simulink library "casper_library"  (Simulink 6.2)
PostLoadFcn:
  | % Stub definitions for mask variables
  | delay_depth=16;
  | n_bits=8;
  | bin_pt=7;
values from neighbouring files (symbols this model uses):
  add_latency = get_var('add_latency', 'defaults', defaults, varargin{:})    [biplex_core_init.m]    (also in butterfly_direct_init.m; dec_fir_init.m = get_var('add_latency','defaults', defaults, varargin{:}); fft_biplex_real_4x_init.m; fft_direct_init.m)
  BitWidth = get_var('BitWidth', 'defaults', defaults, varargin{:})    [biplex_core_init.m]    (also in butterfly_direct_init.m; fft_biplex_init.m; fft_biplex_real_2x_init.m; fft_biplex_real_4x_init.m)
  blockCountBits = ceil(log2(numBlocks))    [address_gen_vacc_v2_mask.m]
  blockRowBits = 0    [address_gen_vacc_v2_mask.m]
  mult_latency = get_var('mult_latency', 'defaults', defaults, varargin{:})    [biplex_core_init.m]    (also in butterfly_direct_init.m; dec_fir_init.m = get_var('mult_latency','defaults', defaults, varargin{:}); fft_biplex_real_4x_init.m; fft_direct_init.m)
  n_inputs = get_var('n_inputs', 'defaults', defaults, varargin{:})    [adder_tree_init.m]    (also in barrel_switcher_init.m; dec_fir_init.m = get_var('n_inputs','defaults', defaults, varargin{:}); fft_init.m; fft_unscrambler_init.m)
undefined symbols (not defined in the file or in its folder): acc_len, ant_bits, bit_growth, bit_rev, BitWidthIn, cmult_4bit_br, cmult_4bit_em, cmult_4bit_sl, CoeffBitWidth, DelayLen, n_ants, n_bits_out, pfb_coeff_gen_calc, PFBSize
libraries: xbsIndex_r3 x2630, casper_library x215, xps_library x24, fft_library x4
(part 3 of 21)

== system casper_library/Delays/delay_bram_prog_dp ==
  din : Inport  Port=1  LatchInput=off
  delay : Inport  Port=2  LatchInput=off
  AddSub : xbsIndex_r3/AddSub  mode=Subtraction  precision=User Defined  arith_type=Unsigned  n_bits=ram_bits  bin_pt=0  quantization=Truncate  overflow=Wrap  latency=1  explicit_period=off  period=1  use_carryin=off  use_carryout=off  en=off  dbl_ovrd=off  show_param=off  use_core=on  pipeline=off  use_rpm=on  gen_core=off
      settings: xl_area=[0, 0, 0, 0, 0, 0, 0]
  Constant2 : xbsIndex_r3/Constant  const=1  equ=P=C  arith_type=Boolean  n_bits=1  bin_pt=0  opselect=C  inp2=PCIN>>17  opr=+  inp1=P  carry=CIN  iostate=0  explicit_period=on  period=1  dbl_ovrd=off
  Constant4 : xbsIndex_r3/Constant  const=0  equ=P=C  arith_type=Boolean  n_bits=1  bin_pt=0  opselect=C  inp2=PCIN>>17  opr=+  inp1=P  carry=CIN  iostate=0  explicit_period=on  period=1  dbl_ovrd=off
  Dual Port RAM : S-Function  AncestorBlock=xbsIndex_r3/Dual Port RAM  FunctionName=xldpram  Parameters=sfcn_mwsv__  mask(Xilinx Dual Port Random Access Memory){depth=2^ram_bits, initVector=0, write_mode_A=Read After Write, write_mode_B=Read After Write, latency=bram_latency, mem_collision=off, init_zero=on, explicit_period=off, period=1, dbl_ovrd=off, rst_a=off, init_a=0, rst_b=off, init_b=0, show_param=off, distributed_mem=off, use_rpm=off, gen_core=off, xl_area=[0, 0, 0, 0, 0, 0, 0], xl_use_area=off}
      mask prompts: initVector "Initial Value Vector"; write_mode_A "Write Mode:  Port A"; write_mode_B "Write Mode:  Port B"; mem_collision "Provide Output Valid Port"; init_zero "Zero Initial Output  (otherwise NaN)"; explicit_period "Use Explicit Sample Period"; period "Sample Period  (use -1 to inherit first known input period)"; dbl_ovrd "Override with Doubles"; rst_a "Provide Reset Port for Port A Output Register"; init_a "Initial Value for Port A Output Register"; rst_b "Provide Reset Port for Port B Output Register"; init_b "Initial Value for Port B Output Register"; show_param "---------------------- Show Implementation Parameters -----------------------------------------------------------------------------------"; distributed_mem "Use Distributed Memory (instead of block RAM)"; use_rpm "Use Placement Information for Core"; gen_core "Generate Core"; xl_area "FPGA Area [Slices, FFs, BRAMs, LUTs, IOBs, Emb. Mults, TBUFs]"; xl_use_area "Use Area Above For Estimation"
      mask help: Dual port random access memory (RAM). Independent address, data and write enable ports allow shared access to a single memory space. Dual ports enable simultaneous access to the memory space at different sample rates using multiple data widths.
      mask init:
      | [designRoot, family, part, speed, package, simulinkPeriod, sysclkPeriod, dbl_ovrd, trimVbit] = xlSysgenSettings(gcb,1,1);
      | if isempty(family)
      | 	family = 'Virtex2';
      | end;
      | dbl_ovrdStr = '';
      | [bg,fg] = xlcmap('XBlock',dbl_ovrd);
      | iPos = get_param(gcb,'Position');
      | iWidth=iPos(3)-iPos(1); iHeight=iPos(4)-iPos(2);
      | iCx=iWidth/2;
      | iCy=iHeight/2;
      | [logoX, logoY] = xlogo(iPos);
      | [memX,memY] = memplot(iPos,min(depth,floor(iWidth/4)));
      | 
      | dataBPNum = 1;
      | dataBStr = '';
      | weBPNum = 1;
      | weBStr = '';
      | rstAPNum = 1;
      | rstAStr = '';
      | rstBPNum = 1;
      | rstBStr = '';
      | if(distributed_mem==0)
      |    dataBPNum = 5;
      |    dataBStr = 'data_B';
      |    weBPNum = 6;
      |    weBStr = 'we_B';
      |    if (latency==1)
      | 	   if (rst_a)
      | 		   rstAPNum = 7;
      | 		   rstAStr = 'rst_A';
      | 		   if (rst_b)
      | 	   			rstBPNum = 8;
      | 				rstBStr = 'rst_B';
      | 			end
      | 		else
      | 			if (rst_b)
      | 	   			rstBPNum = 7;
      | 				rstBStr = 'rst_B';
      | 			end
      | 		end
      |    end
      | end
      | 
      | voutAPNum = 1;
      | voutAStr = '';
      | voutBPNum = 1;
      | voutBStr = '';
      | doutBPNum=2;
      | if((mem_collision==1) && (distributed_mem==0) )
      |    voutAPNum = 2;
      |    voutAStr = 'vout_A';
      |    doutBPNum=3;
      |    voutBPNum = 4;
      |    voutBStr = 'vout_B';
      | end
      | 
      | % one time added for param list
      | useCore = 1;
      | dblOvrd = dbl_ovrd;
      | precision0 = 1;
      | precision1 = 1;
      | precision2 = 1;
      | precision3 = 1;
      | depthA = depth;
      | init = initVector;
      | write_mode_a = write_mode_A;
      | write_mode_b = write_mode_B;
      | initZero = init_zero;
      | explicitClk = explicit_period;
      | gen_core = 1;
      | 
      | % just pass everything to s-function
      | sfcn_mwsv__ = get_param(gcb, 'MaskWSVariables');
      mask Help: eval('xlWeb(xlhtmldoclink(''Dual Port RAM''))');
      mask StyleString: edit,edit,popup(Read After Write|Read Before Write|No Read On Write),popup(Read After Write|Read Before Write|No Read On Write),edit,checkbox,checkbox,checkbox,edit,checkbox,checkbox,edit,checkbox,edit,checkbox,checkbox,checkbox,checkbox,edit,checkbox
      mask CallbackString: |||||||xldpramCallback|||xldpramCallback||xldpramCallback||xldpramCallback|xldpramCallback||||
      mask Display:
      | patch([0 iWidth iWidth 0],[0 0 iHeight iHeight] ,bg);
      | patch([0 iWidth iWidth 0],[iCy-2 iCy-2 iCy+2 iCy+2] , .9* bg);
      | patch(logoX,logoY , fg);
      | port_label('input',1,'addr_A');
      | port_label('input',2,'data_A');
      | port_label('input',3,'we_A');
      | port_label('input',4,'addr_B');
      | port_label('input',dataBPNum,dataBStr);
      | port_label('input',weBPNum,weBStr);
      | port_label('input',rstAPNum,rstAStr);
      | port_label('input',rstBPNum,rstBStr);
      | port_label('output',1,'A');
      | port_label('output',doutBPNum,'B');
      | port_label('output',voutAPNum,voutAStr);
      | port_label('output',voutBPNum,voutBStr);
      | ;plot([0 0 iWidth iWidth 0], [0 iHeight iHeight 0 0]);
  wr_addr : xbsIndex_r3/Counter  cnt_type=Free Running  n_bits=ram_bits  bin_pt=0  arith_type=Unsigned  start_count=0  cnt_to=Inf  cnt_by_val=1  operation=Up  explicit_period=off  period=1  load_pin=off  rst=off  en=off  dbl_ovrd=off  show_param=off  use_rpm=on  gen_core=off
      settings: xl_area=[0, 0, 0, 0, 0, 0, 0]
  dout : Outport
  wires:
  Dual Port RAM/2 -> dout/1
  AddSub/1 -> Dual Port RAM/4
  delay/1 -> AddSub/2
  Constant4/1 -> Dual Port RAM/6
  din/1 -> Dual Port RAM/2, Dual Port RAM/5
  Constant2/1 -> Dual Port RAM/3
  wr_addr/1 -> Dual Port RAM/1, AddSub/1

== system casper_library/Delays/delay_complex ==
  In1 : Inport  Port=1  LatchInput=off
  c_to_ri : casper_library/Misc/c_to_ri  n_bits=18  bin_pt=17
      settings: AttributesFormatString=18_17 r/i
  delay1 : Subsystem  BlockChoice=delay_bram
      link override delay_bram: DelayLen=delay  bram_latency=bram_latency
      link override delay_slr: DelayLen=delay
      settings: AttributesFormatString=%<BlockChoice>  TemplateBlock=casper_library/Delays/delay  MemberBlocks=delay_bram,delay_slr
  delay2 : Subsystem  BlockChoice=delay_bram
      link override delay_bram: DelayLen=delay  bram_latency=bram_latency
      link override delay_slr: DelayLen=delay
      settings: AttributesFormatString=%<BlockChoice>  TemplateBlock=casper_library/Delays/delay  MemberBlocks=delay_bram,delay_slr
  ri_to_c : casper_library/Misc/ri_to_c
  Out1 : Outport
  wires:
  c_to_ri/1 -> delay1/1(In1)
  delay1/1(Out1) -> ri_to_c/1
  c_to_ri/2 -> delay2/1(In1)
  delay2/1(Out1) -> ri_to_c/2
  In1/1 -> c_to_ri/1
  ri_to_c/1 -> Out1/1

== system casper_library/Delays/delay_slr ==
  In1 : Inport  Port=1  LatchInput=off
  delay_slr : xbsIndex_r3/Delay  latency=DelayLen  reg_retiming=off  explicit_period=off  period=1  en=off  accept_only_valid=off  init_zero=on  dbl_ovrd=off  show_param=off
      settings: xl_area=[0, 0, 0, 0, 0, 0, 0]
  Out1 : Outport
  wires:
  delay_slr/1 -> Out1/1
  In1/1 -> delay_slr/1

== system casper_library/Delays/delay_wideband_prog ==
  delay : Inport  Port=1  LatchInput=off
  sync : Inport  Port=2  LatchInput=off
  data_in1 : Inport  Port=3  LatchInput=off
  data_in2 : Inport  Port=4  LatchInput=off
  data_in3 : Inport  Port=5  LatchInput=off
  data_in4 : Inport  Port=6  LatchInput=off
  AddSub1 : xbsIndex_r3/AddSub  mode=Addition  precision=Full  arith_type=Unsigned  n_bits=8  bin_pt=0  quantization=Truncate  overflow=Wrap  latency=0  explicit_period=off  period=1  use_carryin=off  use_carryout=off  en=off  dbl_ovrd=off  show_param=off  use_core=on  pipeline=off  use_rpm=on  gen_core=off
      settings: xl_area=[0, 0, 0, 0, 0, 0, 0]
  AddSub2 : xbsIndex_r3/AddSub  mode=Addition  precision=Full  arith_type=Unsigned  n_bits=8  bin_pt=0  quantization=Truncate  overflow=Wrap  latency=0  explicit_period=off  period=1  use_carryin=off  use_carryout=off  en=off  dbl_ovrd=off  show_param=off  use_core=on  pipeline=off  use_rpm=on  gen_core=off
      settings: xl_area=[0, 0, 0, 0, 0, 0, 0]
  AddSub3 : xbsIndex_r3/AddSub  mode=Addition  precision=Full  arith_type=Unsigned  n_bits=8  bin_pt=0  quantization=Truncate  overflow=Wrap  latency=0  explicit_period=off  period=1  use_carryin=off  use_carryout=off  en=off  dbl_ovrd=off  show_param=off  use_core=on  pipeline=off  use_rpm=on  gen_core=off
      settings: xl_area=[0, 0, 0, 0, 0, 0, 0]
  Constant1 : xbsIndex_r3/Constant  const=2  equ=P=C  arith_type=Unsigned  n_bits=2  bin_pt=0  opselect=C  inp2=PCIN>>17  opr=+  inp1=P  carry=CIN  iostate=0  explicit_period=on  period=1  dbl_ovrd=off
  Constant2 : xbsIndex_r3/Constant  const=1  equ=P=C  arith_type=Unsigned  n_bits=2  bin_pt=0  opselect=C  inp2=PCIN>>17  opr=+  inp1=P  carry=CIN  iostate=0  explicit_period=on  period=1  dbl_ovrd=off
  Constant3 : xbsIndex_r3/Constant  const=0  equ=P=C  arith_type=Unsigned  n_bits=2  bin_pt=0  opselect=C  inp2=PCIN>>17  opr=+  inp1=P  carry=CIN  iostate=0  explicit_period=on  period=1  dbl_ovrd=off
  Convert1 : xbsIndex_r3/Convert  arith_type=Unsigned  n_bits=1  bin_pt=0  quantization=Truncate  overflow=Wrap  latency=0  explicit_period=off  period=1  dbl_ovrd=off  show_param=off  inserted_by_tool=off  pipeline=off
      settings: xl_area=[0, 0, 0, 0, 0, 0, 0]
  Convert2 : xbsIndex_r3/Convert  arith_type=Unsigned  n_bits=1  bin_pt=0  quantization=Truncate  overflow=Wrap  latency=0  explicit_period=off  period=1  dbl_ovrd=off  show_param=off  inserted_by_tool=off  pipeline=off
      settings: xl_area=[0, 0, 0, 0, 0, 0, 0]
  Convert3 : xbsIndex_r3/Convert  arith_type=Unsigned  n_bits=1  bin_pt=0  quantization=Truncate  overflow=Wrap  latency=0  explicit_period=off  period=1  dbl_ovrd=off  show_param=off  inserted_by_tool=off  pipeline=off
      settings: xl_area=[0, 0, 0, 0, 0, 0, 0]
  Relational1 : xbsIndex_r3/Relational  mode=a>b  latency=0  explicit_period=off  period=1  en=off  dbl_ovrd=off  show_param=off
      settings: xl_area=[0, 0, 0, 0, 0, 0, 0]
  Relational2 : xbsIndex_r3/Relational  mode=a>b  latency=0  explicit_period=off  period=1  en=off  dbl_ovrd=off  show_param=off
      settings: xl_area=[0, 0, 0, 0, 0, 0, 0]
  Relational3 : xbsIndex_r3/Relational  mode=a>b  latency=0  explicit_period=off  period=1  en=off  dbl_ovrd=off  show_param=off
      settings: xl_area=[0, 0, 0, 0, 0, 0, 0]
  barrel_switcher : Subsystem  mask(barrel_switcher){n_inputs=2}
      mask prompts: n_inputs "Number of Inputs: (2^?)"
      mask init:
      | barrel_switcher_init(gcb,...
      |     'n_inputs', n_inputs);
      settings: AttributesFormatString=n_inputs=2
  bram_rd_addrs : xbsIndex_r3/Slice  mode=Lower Bit Location + Width  nbits=8  bit1=0  base1=MSB of Input  bit0=2  base0=LSB of Input  boolean_output=off  explicit_period=off  period=1  dbl_ovrd=off
  bs_sel : xbsIndex_r3/Slice  mode=Lower Bit Location + Width  nbits=2  bit1=0  base1=MSB of Input  bit0=0  base0=LSB of Input  boolean_output=off  explicit_period=off  period=1  dbl_ovrd=off
  delay_dp : Subsystem  mask{ram_bits=8, bram_latency=4}
      mask prompts: ram_bits "Max Delay (2^?)"; bram_latency "BRAM Latency"
  delay_dp1 : Subsystem  mask{ram_bits=8, bram_latency=4}
      mask prompts: ram_bits "Max Delay (2^?)"; bram_latency "BRAM Latency"
  delay_dp2 : Subsystem  mask{ram_bits=8, bram_latency=4}
      mask prompts: ram_bits "Max Delay (2^?)"; bram_latency "BRAM Latency"
  delay_dp3 : Subsystem  mask{ram_bits=8, bram_latency=4}
      mask prompts: ram_bits "Max Delay (2^?)"; bram_latency "BRAM Latency"
  delay_reg : xbsIndex_r3/Register  init=0  reg_only_valid=off  explicit_period=off  period=1  rst=off  en=on  out_en=off  dbl_ovrd=off  show_param=off
      settings: xl_area=[0, 0, 0, 0, 0, 0, 0]
  delay_sel : xbsIndex_r3/Delay  latency=5  reg_retiming=off  explicit_period=off  period=1  en=off  accept_only_valid=off  init_zero=on  dbl_ovrd=off  show_param=off
      settings: xl_area=[0, 0, 0, 0, 0, 0, 0]
  max_delay : xbsIndex_r3/Constant  const=1023  equ=P=C  arith_type=Unsigned  n_bits=32  bin_pt=0  opselect=C  inp2=PCIN>>17  opr=+  inp1=P  carry=CIN  iostate=0  explicit_period=on  period=1  dbl_ovrd=off
  max_delay_chk : xbsIndex_r3/Relational  mode=a<=b  latency=1  explicit_period=off  period=1  en=off  dbl_ovrd=off  show_param=off
      settings: xl_area=[0, 0, 0, 0, 0, 0, 0]
  mux_delay : xbsIndex_r3/Mux  inputs=2  precision=Full  arith_type="Signed  (2's comp)"  n_bits=8  bin_pt=2  quantization=Truncate  overflow=Wrap  latency=0  explicit_period=off  period=1  en=off  dbl_ovrd=off  show_param=off  mux_type=off  use_rpm=off  gen_core=off
      settings: xl_area=[0, 0, 0, 0, 0, 0, 0]
  sync_delay : Subsystem  mask(sync_delay){DelayLen=5}
      mask prompts: DelayLen "Delay Length:"
      mask help: Delay an infrequent boolean pulse by the specified number of clocks.
      mask init:
      | BitWidth = max(2, ceil(log2(DelayLen+1)));
      | UseCounter = 1;
      | if DelayLen == 0,
      | 	UseCounter = 0;
      | end
      mask Help: eval('xlWeb([getenv(''MLIB_ROOT''), ''\casper_library\doc\sync_delay_usage.html''])')
      mask Display: fprintf('Z^-%d', DelayLen)
  sync_out : Outport
  data_out1 : Outport  Port=2
  data_out2 : Outport  Port=3
  data_out3 : Outport  Port=4
  data_out4 : Outport  Port=5
  wires:
  delay/1 -> delay_reg/1
  delay_reg/1 -> max_delay_chk/1, mux_delay/3
  sync/1 -> delay_reg/2, sync_delay/1(In)
  max_delay/1 -> max_delay_chk/2, mux_delay/2
  max_delay_chk/1 -> mux_delay/1
  data_in1/1 -> delay_dp/1(din)
  bram_rd_addrs/1 -> delay_dp/2(delay), AddSub1/1, AddSub2/1, AddSub3/1
  mux_delay/1 -> bram_rd_addrs/1, bs_sel/1
  bs_sel/1 -> Relational1/1, Relational2/1, Relational3/1, delay_sel/1
  Constant1/1 -> Relational1/2
  Relational1/1 -> Convert1/1
  Convert1/1 -> AddSub1/2
  barrel_switcher/2(Out1) -> data_out4/1
  AddSub1/1 -> delay_dp1/2(delay)
  data_in2/1 -> delay_dp1/1(din)
  delay_dp1/1(dout) -> barrel_switcher/5(In3)
  Constant2/1 -> Relational2/2
  Relational2/1 -> Convert2/1
  Convert2/1 -> AddSub2/2
  barrel_switcher/3(Out2) -> data_out3/1
  AddSub2/1 -> delay_dp2/2(delay)
  data_in3/1 -> delay_dp2/1(din)
  delay_dp2/1(dout) -> barrel_switcher/4(In2)
  Constant3/1 -> Relational3/2
  Relational3/1 -> Convert3/1
  Convert3/1 -> AddSub3/2
  barrel_switcher/4(Out3) -> data_out2/1
  AddSub3/1 -> delay_dp3/2(delay)
  data_in4/1 -> delay_dp3/1(din)
  delay_dp3/1(dout) -> barrel_switcher/3(In1)
  delay_sel/1 -> barrel_switcher/1(sel)
  barrel_switcher/1(sync_out) -> sync_out/1
  barrel_switcher/5(Out4) -> data_out1/1
  sync_delay/1(Out) -> barrel_switcher/2(sync_in)
  delay_dp/1(dout) -> barrel_switcher/6(In4)

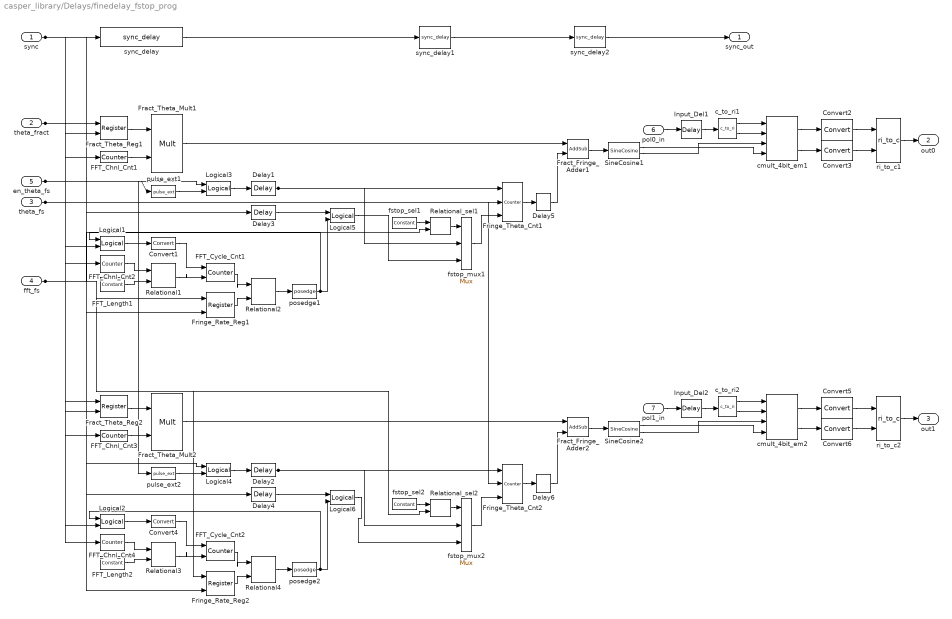
== system casper_library/Delays/finedelay_fstop_prog ==
  sync : Inport  Port=1  LatchInput=off
  theta_fract : Inport  Port=2  LatchInput=off
  theta_fs : Inport  Port=3  LatchInput=off
  fft_fs : Inport  Port=4  LatchInput=off
  en_theta_fs : Inport  Port=5  LatchInput=off
  pol0_in : Inport  Port=6  LatchInput=off
  pol1_in : Inport  Port=7  LatchInput=off
  Convert1 : xbsIndex_r3/Convert  arith_type=Boolean  n_bits=8  bin_pt=6  quantization=Truncate  overflow=Wrap  latency=0  explicit_period=on  period=1  dbl_ovrd=off  show_param=off  inserted_by_tool=off  pipeline=off
      settings: xl_area=[0, 0, 0, 0, 0, 0, 0]
  Convert{2..3,5..6} (4 alike) : xbsIndex_r3/Convert  arith_type="Signed  (2's comp)"  n_bits=fft_bits  bin_pt=fft_bits-1  quantization=Truncate  overflow=Wrap  latency=0  explicit_period=off  period=1  dbl_ovrd=off  show_param=off  inserted_by_tool=off  pipeline=off
      settings: xl_area=[0, 0, 0, 0, 0, 0, 0]
  Convert4 : xbsIndex_r3/Convert  arith_type=Boolean  n_bits=8  bin_pt=6  quantization=Truncate  overflow=Wrap  latency=0  explicit_period=on  period=1  dbl_ovrd=off  show_param=off  inserted_by_tool=off  pipeline=off
      settings: xl_area=[0, 0, 0, 0, 0, 0, 0]
  Delay{1..4} (4 alike) : xbsIndex_r3/Delay  latency=1  reg_retiming=off  explicit_period=off  period=1  en=off  accept_only_valid=off  init_zero=on  dbl_ovrd=off  show_param=off
      settings: xl_area=[0, 0, 0, 0, 0, 0, 0]
  Delay5 : xbsIndex_r3/Delay  latency=2  reg_retiming=off  explicit_period=off  period=1  en=off  accept_only_valid=off  init_zero=on  dbl_ovrd=off  show_param=off
      settings: xl_area=[0, 0, 0, 0, 0, 0, 0]
  Delay6 : xbsIndex_r3/Delay  latency=2  reg_retiming=off  explicit_period=off  period=1  en=off  accept_only_valid=off  init_zero=on  dbl_ovrd=off  show_param=off
      settings: xl_area=[0, 0, 0, 0, 0, 0, 0]
  FFT_Chnl_Cnt1 : xbsIndex_r3/Counter  cnt_type=Free Running  n_bits=10  bin_pt=0  arith_type=Unsigned  start_count=0  cnt_to=Inf  cnt_by_val=2  operation=Up  explicit_period=off  period=1  load_pin=off  rst=on  en=off  dbl_ovrd=off  show_param=off  use_rpm=on  gen_core=off
      settings: xl_area=[0, 0, 0, 0, 0, 0, 0]
  FFT_Chnl_Cnt2 : xbsIndex_r3/Counter  cnt_type=Free Running  n_bits=9  bin_pt=0  arith_type=Unsigned  start_count=0  cnt_to=Inf  cnt_by_val=1  operation=Up  explicit_period=off  period=1  load_pin=off  rst=on  en=off  dbl_ovrd=off  show_param=off  use_rpm=on  gen_core=off
      settings: xl_area=[0, 0, 0, 0, 0, 0, 0]
  FFT_Chnl_Cnt3 : xbsIndex_r3/Counter  cnt_type=Free Running  n_bits=10  bin_pt=0  arith_type=Unsigned  start_count=1  cnt_to=Inf  cnt_by_val=2  operation=Up  explicit_period=off  period=1  load_pin=off  rst=on  en=off  dbl_ovrd=off  show_param=off  use_rpm=on  gen_core=off
      settings: xl_area=[0, 0, 0, 0, 0, 0, 0]
  FFT_Chnl_Cnt4 : xbsIndex_r3/Counter  cnt_type=Free Running  n_bits=9  bin_pt=0  arith_type=Unsigned  start_count=0  cnt_to=Inf  cnt_by_val=1  operation=Up  explicit_period=off  period=1  load_pin=off  rst=on  en=off  dbl_ovrd=off  show_param=off  use_rpm=on  gen_core=off
      settings: xl_area=[0, 0, 0, 0, 0, 0, 0]
  FFT_Cycle_Cnt1 : xbsIndex_r3/Counter  cnt_type=Free Running  n_bits=17  bin_pt=0  arith_type=Unsigned  start_count=0  cnt_to=Inf  cnt_by_val=1  operation=Up  explicit_period=off  period=1  load_pin=off  rst=on  en=on  dbl_ovrd=off  show_param=off  use_rpm=on  gen_core=off
      settings: xl_area=[0, 0, 0, 0, 0, 0, 0]
  FFT_Cycle_Cnt2 : xbsIndex_r3/Counter  cnt_type=Free Running  n_bits=17  bin_pt=0  arith_type=Unsigned  start_count=0  cnt_to=Inf  cnt_by_val=1  operation=Up  explicit_period=off  period=1  load_pin=off  rst=on  en=on  dbl_ovrd=off  show_param=off  use_rpm=on  gen_core=off
      settings: xl_area=[0, 0, 0, 0, 0, 0, 0]
  FFT_Length1 : xbsIndex_r3/Constant  const=511  equ=P=C  arith_type=Unsigned  n_bits=9  bin_pt=0  opselect=C  inp2=PCIN>>17  opr=+  inp1=P  carry=CIN  iostate=0  explicit_period=on  period=1  dbl_ovrd=off
  FFT_Length2 : xbsIndex_r3/Constant  const=511  equ=P=C  arith_type=Unsigned  n_bits=9  bin_pt=0  opselect=C  inp2=PCIN>>17  opr=+  inp1=P  carry=CIN  iostate=0  explicit_period=on  period=1  dbl_ovrd=off
  Fract_Fringe_Adder1 : xbsIndex_r3/AddSub  mode=Addition  precision=User Defined  arith_type=Unsigned  n_bits=14  bin_pt=0  quantization=Truncate  overflow=Wrap  latency=2  explicit_period=off  period=1  use_carryin=off  use_carryout=off  en=off  dbl_ovrd=off  show_param=off  use_core=on  pipeline=off  use_rpm=on  gen_core=off
      settings: xl_area=[0, 0, 0, 0, 0, 0, 0]
  Fract_Fringe_Adder2 : xbsIndex_r3/AddSub  mode=Addition  precision=User Defined  arith_type=Unsigned  n_bits=14  bin_pt=0  quantization=Truncate  overflow=Wrap  latency=2  explicit_period=off  period=1  use_carryin=off  use_carryout=off  en=off  dbl_ovrd=off  show_param=off  use_core=on  pipeline=off  use_rpm=on  gen_core=off
      settings: xl_area=[0, 0, 0, 0, 0, 0, 0]
  Fract_Theta_Mult1 : xbsIndex_r3/Mult  precision=User Defined  arith_type=Unsigned  n_bits=14  bin_pt=0  quantization=Truncate  overflow=Wrap  latency=3  explicit_period=off  period=1  en=off  dbl_ovrd=off  show_param=on  mult_type=Parallel  oversample=2  use_embedded=on  pipeline=on  use_rpm=on  placement_style=Rectangular Shape  gen_core=off
      settings: xl_area=[0, 0, 0, 0, 0, 0, 0]
  Fract_Theta_Mult2 : xbsIndex_r3/Mult  precision=User Defined  arith_type=Unsigned  n_bits=14  bin_pt=0  quantization=Truncate  overflow=Wrap  latency=3  explicit_period=off  period=1  en=off  dbl_ovrd=off  show_param=on  mult_type=Parallel  oversample=2  use_embedded=on  pipeline=on  use_rpm=on  placement_style=Rectangular Shape  gen_core=off
      settings: xl_area=[0, 0, 0, 0, 0, 0, 0]
  Fract_Theta_Reg1 : xbsIndex_r3/Register  init=0  reg_only_valid=off  explicit_period=off  period=1  rst=off  en=on  out_en=off  dbl_ovrd=off  show_param=off
      settings: xl_area=[0, 0, 0, 0, 0, 0, 0]
  Fract_Theta_Reg2 : xbsIndex_r3/Register  init=0  reg_only_valid=off  explicit_period=off  period=1  rst=off  en=on  out_en=off  dbl_ovrd=off  show_param=off
      settings: xl_area=[0, 0, 0, 0, 0, 0, 0]
  Fringe_Rate_Reg1 : xbsIndex_r3/Register  init=0  reg_only_valid=off  explicit_period=off  period=1  rst=off  en=on  out_en=off  dbl_ovrd=off  show_param=off
      settings: xl_area=[0, 0, 0, 0, 0, 0, 0]
  Fringe_Rate_Reg2 : xbsIndex_r3/Register  init=0  reg_only_valid=off  explicit_period=off  period=1  rst=off  en=on  out_en=off  dbl_ovrd=off  show_param=off
      settings: xl_area=[0, 0, 0, 0, 0, 0, 0]
  Fringe_Theta_Cnt1 : xbsIndex_r3/Counter  cnt_type=Free Running  n_bits=14  bin_pt=0  arith_type=Unsigned  start_count=0  cnt_to=Inf  cnt_by_val=1  operation=Up  explicit_period=on  period=1  load_pin=on  rst=off  en=on  dbl_ovrd=off  show_param=off  use_rpm=on  gen_core=off
      settings: xl_area=[0, 0, 0, 0, 0, 0, 0]
  Fringe_Theta_Cnt2 : xbsIndex_r3/Counter  cnt_type=Free Running  n_bits=14  bin_pt=0  arith_type=Unsigned  start_count=0  cnt_to=Inf  cnt_by_val=1  operation=Up  explicit_period=on  period=1  load_pin=on  rst=off  en=on  dbl_ovrd=off  show_param=off  use_rpm=on  gen_core=off
      settings: xl_area=[0, 0, 0, 0, 0, 0, 0]
  Input_Del1 : xbsIndex_r3/Delay  latency=7  reg_retiming=off  explicit_period=off  period=1  en=off  accept_only_valid=off  init_zero=on  dbl_ovrd=off  show_param=off
      settings: xl_area=[0, 0, 0, 0, 0, 0, 0]
  Input_Del2 : xbsIndex_r3/Delay  latency=7  reg_retiming=off  explicit_period=off  period=1  en=off  accept_only_valid=off  init_zero=on  dbl_ovrd=off  show_param=off
      settings: xl_area=[0, 0, 0, 0, 0, 0, 0]
  Logical{1..2,5..6} (4 alike) : xbsIndex_r3/Logical  logical_function=OR  inputs=2  precision=Full  arith_type=Unsigned  n_bits=1  bin_pt=0  align_bp=on  latency=0  explicit_period=on  period=1  en=off  dbl_ovrd=off  show_param=off
      settings: xl_area=[0, 0, 0, 0, 0, 0, 0]
  Logical3 : xbsIndex_r3/Logical  logical_function=AND  inputs=2  precision=Full  arith_type=Unsigned  n_bits=1  bin_pt=0  align_bp=on  latency=0  explicit_period=on  period=1  en=off  dbl_ovrd=off  show_param=off
      settings: xl_area=[0, 0, 0, 0, 0, 0, 0]
  Logical4 : xbsIndex_r3/Logical  logical_function=AND  inputs=2  precision=Full  arith_type=Unsigned  n_bits=1  bin_pt=0  align_bp=on  latency=0  explicit_period=on  period=1  en=off  dbl_ovrd=off  show_param=off
      settings: xl_area=[0, 0, 0, 0, 0, 0, 0]
  Relational{1..4} (4 alike) : xbsIndex_r3/Relational  mode=a=b  latency=0  explicit_period=off  period=1  en=off  dbl_ovrd=off  show_param=off
      settings: xl_area=[0, 0, 0, 0, 0, 0, 0]
  Relational_sel1 : xbsIndex_r3/Relational  mode=a!=b  latency=0  explicit_period=off  period=1  en=off  dbl_ovrd=off  show_param=off
      settings: xl_area=[0, 0, 0, 0, 0, 0, 0]
  Relational_sel2 : xbsIndex_r3/Relational  mode=a!=b  latency=0  explicit_period=off  period=1  en=off  dbl_ovrd=off  show_param=off
      settings: xl_area=[0, 0, 0, 0, 0, 0, 0]
  SineCosine1 : xbsIndex_r3/SineCosine  mode=Sine and Cosine  neg_sin=off  neg_cos=off  n_bits=18  latency=2  sym_output=off  explicit_period=off  period=1  en=off  dbl_ovrd=off  show_param=on  mem_type=Block RAM  pipeline=off  use_rpm=on  gen_core=off
      settings: xl_area=[0, 0, 0, 0, 0, 0, 0]
  SineCosine2 : xbsIndex_r3/SineCosine  mode=Sine and Cosine  neg_sin=off  neg_cos=off  n_bits=18  latency=2  sym_output=off  explicit_period=off  period=1  en=off  dbl_ovrd=off  show_param=on  mem_type=Block RAM  pipeline=off  use_rpm=on  gen_core=off
      settings: xl_area=[0, 0, 0, 0, 0, 0, 0]
  c_to_ri1 : casper_library/Misc/c_to_ri  n_bits=18  bin_pt=17
      settings: AttributesFormatString=18_17 r/i
  c_to_ri2 : casper_library/Misc/c_to_ri  n_bits=18  bin_pt=17
      settings: AttributesFormatString=18_17 r/i
  cmult_4bit_em1 : casper_library/Multipliers/cmult_4bit_em  mult_latency=2  add_latency=0
  cmult_4bit_em2 : casper_library/Multipliers/cmult_4bit_em  mult_latency=2  add_latency=0
  fstop_mux1 : xbsIndex_r3/Mux  inputs=2  precision=Full  arith_type="Signed  (2's comp)"  n_bits=8  bin_pt=2  quantization=Truncate  overflow=Wrap  latency=0  explicit_period=off  period=1  en=off  dbl_ovrd=off  show_param=off  mux_type=off  use_rpm=off  gen_core=off
      settings: xl_area=[0, 0, 0, 0, 0, 0, 0]
  fstop_mux2 : xbsIndex_r3/Mux  inputs=2  precision=Full  arith_type="Signed  (2's comp)"  n_bits=8  bin_pt=2  quantization=Truncate  overflow=Wrap  latency=0  explicit_period=off  period=1  en=off  dbl_ovrd=off  show_param=off  mux_type=off  use_rpm=off  gen_core=off
      settings: xl_area=[0, 0, 0, 0, 0, 0, 0]
  fstop_sel1 : xbsIndex_r3/Constant  const=0  equ=P=C  arith_type=Unsigned  n_bits=17  bin_pt=0  opselect=C  inp2=PCIN>>17  opr=+  inp1=P  carry=CIN  iostate=0  explicit_period=on  period=1  dbl_ovrd=off
  fstop_sel2 : xbsIndex_r3/Constant  const=0  equ=P=C  arith_type=Unsigned  n_bits=17  bin_pt=0  opselect=C  inp2=PCIN>>17  opr=+  inp1=P  carry=CIN  iostate=0  explicit_period=on  period=1  dbl_ovrd=off
  posedge1 : casper_library/Misc/posedge  Tag=Rising Edge Detector
  posedge2 : casper_library/Misc/posedge  Tag=Rising Edge Detector
  pulse_ext1 : casper_library/Misc/pulse_ext  pulse_len=2^27
  pulse_ext2 : casper_library/Misc/pulse_ext  pulse_len=2^27
  ri_to_c1 : casper_library/Misc/ri_to_c
  ri_to_c2 : casper_library/Misc/ri_to_c
  sync_delay : casper_library/Delays/sync_delay  DelayLen=3
  sync_delay1 : casper_library/Delays/sync_delay  DelayLen=4
  sync_delay2 : casper_library/Delays/sync_delay  DelayLen=2
  sync_out : Outport
  out0 : Outport  Port=2
  out1 : Outport  Port=3
  wires:
  sync/1 -> sync_delay/1, Fract_Theta_Reg1/2, FFT_Chnl_Cnt1/1, Logical3/1, Logical1/2, FFT_Chnl_Cnt2/1, Fringe_Rate_Reg1/2, Delay3/1, Fract_Theta_Reg2/2, FFT_Chnl_Cnt3/1, Logical4/1, Logical2/2, FFT_Chnl_Cnt4/1, Fringe_Rate_Reg2/2, Delay4/1
  sync_delay/1 -> sync_delay1/1
  sync_delay1/1 -> sync_delay2/1
  sync_delay2/1 -> sync_out/1
  theta_fract/1 -> Fract_Theta_Reg1/1, Fract_Theta_Reg2/1
  Fract_Theta_Reg1/1 -> Fract_Theta_Mult1/1
  FFT_Chnl_Cnt1/1 -> Fract_Theta_Mult1/2
  en_theta_fs/1 -> pulse_ext1/1, pulse_ext2/1
  posedge1/1 -> Logical1/1, Logical5/2
  Logical1/1 -> Convert1/1
  FFT_Chnl_Cnt2/1 -> Relational1/1
  FFT_Length1/1 -> Relational1/2
  Convert1/1 -> FFT_Cycle_Cnt1/1
  Relational1/1 -> FFT_Cycle_Cnt1/2
  fft_fs/1 -> Fringe_Rate_Reg1/1, Relational_sel1/2, Fringe_Rate_Reg2/1, Relational_sel2/2
  FFT_Cycle_Cnt1/1 -> Relational2/1
  Fringe_Rate_Reg1/1 -> Relational2/2
  Relational2/1 -> posedge1/1
  pulse_ext1/1 -> Logical3/2
  Logical3/1 -> Delay1/1
  Delay1/1 -> Fringe_Theta_Cnt1/1, fstop_mux1/2
  theta_fs/1 -> Fringe_Theta_Cnt1/2, Fringe_Theta_Cnt2/2
  Delay3/1 -> Logical5/1
  fstop_sel1/1 -> Relational_sel1/1
  Relational_sel1/1 -> fstop_mux1/1
  Logical5/1 -> fstop_mux1/3
  fstop_mux1/1 -> Fringe_Theta_Cnt1/3
  Fract_Theta_Mult1/1 -> Fract_Fringe_Adder1/1
  Fringe_Theta_Cnt1/1 -> Delay5/1
  Delay5/1 -> Fract_Fringe_Adder1/2
  Fract_Fringe_Adder1/1 -> SineCosine1/1
  pol0_in/1 -> Input_Del1/1
  Input_Del1/1 -> c_to_ri1/1
  c_to_ri1/1 -> cmult_4bit_em1/1
  c_to_ri1/2 -> cmult_4bit_em1/2
  SineCosine1/2 -> cmult_4bit_em1/3
  SineCosine1/1 -> cmult_4bit_em1/4
  cmult_4bit_em1/1 -> Convert2/1
  cmult_4bit_em1/2 -> Convert3/1
  Convert2/1 -> ri_to_c1/1
  Convert3/1 -> ri_to_c1/2
  ri_to_c1/1 -> out0/1
  Fract_Theta_Reg2/1 -> Fract_Theta_Mult2/1
  FFT_Chnl_Cnt3/1 -> Fract_Theta_Mult2/2
  posedge2/1 -> Logical2/1, Logical6/2
  Logical2/1 -> Convert4/1
  FFT_Chnl_Cnt4/1 -> Relational3/1
  FFT_Length2/1 -> Relational3/2
  Convert4/1 -> FFT_Cycle_Cnt2/1
  Relational3/1 -> FFT_Cycle_Cnt2/2
  FFT_Cycle_Cnt2/1 -> Relational4/1
  Fringe_Rate_Reg2/1 -> Relational4/2
  Relational4/1 -> posedge2/1
  pulse_ext2/1 -> Logical4/2
  Logical4/1 -> Delay2/1
  Delay2/1 -> Fringe_Theta_Cnt2/1, fstop_mux2/2
  Delay4/1 -> Logical6/1
  fstop_sel2/1 -> Relational_sel2/1
  Relational_sel2/1 -> fstop_mux2/1
  Logical6/1 -> fstop_mux2/3
  fstop_mux2/1 -> Fringe_Theta_Cnt2/3
  Fract_Theta_Mult2/1 -> Fract_Fringe_Adder2/1
  Fringe_Theta_Cnt2/1 -> Delay6/1
  Delay6/1 -> Fract_Fringe_Adder2/2
  Fract_Fringe_Adder2/1 -> SineCosine2/1
  pol1_in/1 -> Input_Del2/1
  Input_Del2/1 -> c_to_ri2/1
  c_to_ri2/1 -> cmult_4bit_em2/1
  c_to_ri2/2 -> cmult_4bit_em2/2
  SineCosine2/2 -> cmult_4bit_em2/3
  SineCosine2/1 -> cmult_4bit_em2/4
  cmult_4bit_em2/1 -> Convert5/1
  cmult_4bit_em2/2 -> Convert6/1
  Convert5/1 -> ri_to_c2/1
  Convert6/1 -> ri_to_c2/2
  ri_to_c2/1 -> out1/1

== system casper_library/Delays/partial_delay_prog ==
  delay : Inport  Port=1  LatchInput=off
  In1 : Inport  Port=2  LatchInput=off
  In2 : Inport  Port=3  LatchInput=off
  In3 : Inport  Port=4  LatchInput=off
  In4 : Inport  Port=5  LatchInput=off
  Delay{1..4} (4 alike) : xbsIndex_r3/Delay  latency=1  reg_retiming=off  explicit_period=off  period=1  en=off  accept_only_valid=off  init_zero=on  dbl_ovrd=off  show_param=off
      settings: xl_area=[0, 0, 0, 0, 0, 0, 0]
  Mux{1..4} (4 alike) : xbsIndex_r3/Mux  inputs=4  precision=Full  arith_type="Signed  (2's comp)"  n_bits=8  bin_pt=2  quantization=Truncate  overflow=Wrap  latency=2  explicit_period=off  period=1  en=off  dbl_ovrd=off  show_param=off  mux_type=off  use_rpm=off  gen_core=off
      settings: xl_area=[0, 0, 0, 0, 0, 0, 0]
  Out1 : Outport
  Out2 : Outport  Port=2
  Out3 : Outport  Port=3
  Out4 : Outport  Port=4
  wires:
  In1/1 -> Delay1/1, Mux2/5, Mux3/4, Mux4/3
  Mux1/1 -> Out1/1
  delay/1 -> Mux1/1, Mux2/1, Mux3/1, Mux4/1
  Delay1/1 -> Mux1/2
  In2/1 -> Delay2/1, Mux3/5, Mux4/4
  Mux2/1 -> Out2/1
  Delay2/1 -> Mux2/2, Mux1/3
  In3/1 -> Delay3/1, Mux4/5
  Mux3/1 -> Out3/1
  Delay3/1 -> Mux3/2, Mux1/4, Mux2/3
  In4/1 -> Delay4/1
  Mux4/1 -> Out4/1
  Delay4/1 -> Mux4/2, Mux1/5, Mux2/4, Mux3/3

== system casper_library/Delays/sync_delay ==
  In : Inport  Port=1  LatchInput=off
  Constant : xbsIndex_r3/Constant  const=1  equ=P=C  arith_type=Unsigned  n_bits=BitWidth  bin_pt=0  opselect=C  inp2=PCIN>>17  opr=+  inp1=P  carry=CIN  iostate=0  explicit_period=on  period=1  dbl_ovrd=off
  Constant1 : xbsIndex_r3/Constant  const=0  equ=P=C  arith_type=Unsigned  n_bits=BitWidth  bin_pt=0  opselect=C  inp2=PCIN>>17  opr=+  inp1=P  carry=CIN  iostate=0  explicit_period=on  period=1  dbl_ovrd=off
  Constant2 : xbsIndex_r3/Constant  const=DelayLen  equ=P=C  arith_type=Unsigned  n_bits=BitWidth  bin_pt=0  opselect=C  inp2=PCIN>>17  opr=+  inp1=P  carry=CIN  iostate=0  explicit_period=on  period=1  dbl_ovrd=off
  Constant3 : xbsIndex_r3/Constant  const=UseCounter  equ=P=C  arith_type=Unsigned  n_bits=1  bin_pt=0  opselect=C  inp2=PCIN>>17  opr=+  inp1=P  carry=CIN  iostate=0  explicit_period=on  period=1  dbl_ovrd=off
  Counter : xbsIndex_r3/Counter  cnt_type=Free Running  n_bits=BitWidth  bin_pt=0  arith_type=Unsigned  start_count=0  cnt_to=Inf  cnt_by_val=1  operation=Down  explicit_period=on  period=1  load_pin=on  rst=off  en=on  dbl_ovrd=off  show_param=off  use_rpm=on  gen_core=off
      settings: xl_area=[0, 0, 0, 0, 0, 0, 0]
  Logical : xbsIndex_r3/Logical  logical_function=OR  inputs=2  precision=Full  arith_type=Unsigned  n_bits=8  bin_pt=2  align_bp=on  latency=0  explicit_period=on  period=1  en=off  dbl_ovrd=off  show_param=off
      settings: xl_area=[0, 0, 0, 0, 0, 0, 0]
  Mux : xbsIndex_r3/Mux  inputs=2  precision=Full  arith_type="Signed  (2's comp)"  n_bits=8  bin_pt=2  quantization=Truncate  overflow=Wrap  latency=0  explicit_period=off  period=1  en=off  dbl_ovrd=off  show_param=off  mux_type=off  use_rpm=off  gen_core=off
      settings: xl_area=[0, 0, 0, 0, 0, 0, 0]
  Relational : xbsIndex_r3/Relational  mode=a=b  latency=0  explicit_period=off  period=1  en=off  dbl_ovrd=off  show_param=off
      settings: xl_area=[0, 0, 0, 0, 0, 0, 0]
  Relational1 : xbsIndex_r3/Relational  mode=a!=b  latency=0  explicit_period=on  period=1  en=off  dbl_ovrd=off  show_param=off
      settings: xl_area=[0, 0, 0, 0, 0, 0, 0]
  Out : Outport
  wires:
  Mux/1 -> Out/1
  Constant3/1 -> Mux/1
  Relational/1 -> Mux/3
  Relational1/1 -> Logical/2
  Logical/1 -> Counter/3
  In/1 -> Mux/2, Logical/1, Counter/1
  Constant2/1 -> Counter/2
  Constant/1 -> Relational/1
  Constant1/1 -> Relational1/2
  Counter/1 -> Relational/2, Relational1/1

== system casper_library/Delays/sync_delay_en ==
  In : Inport  Port=1  LatchInput=off
  en : Inport  Port=2  LatchInput=off
  Constant : xbsIndex_r3/Constant  const=1  equ=P=C  arith_type=Unsigned  n_bits=BitWidth  bin_pt=0  opselect=C  inp2=PCIN>>17  opr=+  inp1=P  carry=CIN  iostate=0  explicit_period=on  period=1  dbl_ovrd=off
  Constant1 : xbsIndex_r3/Constant  const=0  equ=P=C  arith_type=Unsigned  n_bits=BitWidth  bin_pt=0  opselect=C  inp2=PCIN>>17  opr=+  inp1=P  carry=CIN  iostate=0  explicit_period=on  period=1  dbl_ovrd=off
  Constant2 : xbsIndex_r3/Constant  const=DelayLen  equ=P=C  arith_type=Unsigned  n_bits=BitWidth  bin_pt=0  opselect=C  inp2=PCIN>>17  opr=+  inp1=P  carry=CIN  iostate=0  explicit_period=on  period=1  dbl_ovrd=off
  Constant3 : xbsIndex_r3/Constant  const=UseCounter  equ=P=C  arith_type=Unsigned  n_bits=1  bin_pt=0  opselect=C  inp2=PCIN>>17  opr=+  inp1=P  carry=CIN  iostate=0  explicit_period=on  period=1  dbl_ovrd=off
  Counter : xbsIndex_r3/Counter  cnt_type=Free Running  n_bits=BitWidth  bin_pt=0  arith_type=Unsigned  start_count=0  cnt_to=Inf  cnt_by_val=1  operation=Down  explicit_period=on  period=1  load_pin=on  rst=off  en=on  dbl_ovrd=off  show_param=off  use_rpm=on  gen_core=off
      settings: xl_area=[0, 0, 0, 0, 0, 0, 0]
  Logical : xbsIndex_r3/Logical  logical_function=OR  inputs=2  precision=Full  arith_type=Unsigned  n_bits=8  bin_pt=2  align_bp=on  latency=0  explicit_period=on  period=1  en=off  dbl_ovrd=off  show_param=off
      settings: xl_area=[0, 0, 0, 0, 0, 0, 0]
  Logical1 : xbsIndex_r3/Logical  logical_function=AND  inputs=2  precision=Full  arith_type=Unsigned  n_bits=8  bin_pt=2  align_bp=on  latency=0  explicit_period=on  period=1  en=off  dbl_ovrd=off  show_param=off
      settings: xl_area=[0, 0, 0, 0, 0, 0, 0]
  Mux : xbsIndex_r3/Mux  inputs=2  precision=Full  arith_type="Signed  (2's comp)"  n_bits=8  bin_pt=2  quantization=Truncate  overflow=Wrap  latency=0  explicit_period=off  period=1  en=off  dbl_ovrd=off  show_param=off  mux_type=off  use_rpm=off  gen_core=off
      settings: xl_area=[0, 0, 0, 0, 0, 0, 0]
  Relational : xbsIndex_r3/Relational  mode=a=b  latency=0  explicit_period=off  period=1  en=off  dbl_ovrd=off  show_param=off
      settings: xl_area=[0, 0, 0, 0, 0, 0, 0]
  Relational1 : xbsIndex_r3/Relational  mode=a!=b  latency=0  explicit_period=on  period=1  en=off  dbl_ovrd=off  show_param=off
      settings: xl_area=[0, 0, 0, 0, 0, 0, 0]
  Out : Outport
  wires:
  Counter/1 -> Relational1/1, Relational/2
  Constant1/1 -> Relational1/2
  Constant/1 -> Relational/1
  Constant2/1 -> Counter/2
  In/1 -> Counter/1, Logical/1, Mux/2
  Relational1/1 -> Logical/2
  Relational/1 -> Mux/3
  Constant3/1 -> Mux/1
  Mux/1 -> Out/1
  Logical/1 -> Logical1/1
  Logical1/1 -> Counter/3
  en/1 -> Logical1/2

== system casper_library/Delays/sync_delay_prog ==
  sync : Inport  Port=1  LatchInput=off
  delay : Inport  Port=2  LatchInput=off
  Constant : xbsIndex_r3/Constant  const=1  equ=P=C  arith_type=Unsigned  n_bits=MaxDelay  bin_pt=0  opselect=C  inp2=PCIN>>17  opr=+  inp1=P  carry=CIN  iostate=0  explicit_period=on  period=1  dbl_ovrd=off
  Constant1 : xbsIndex_r3/Constant  const=0  equ=P=C  arith_type=Unsigned  n_bits=MaxDelay  bin_pt=0  opselect=C  inp2=PCIN>>17  opr=+  inp1=P  carry=CIN  iostate=0  explicit_period=on  period=1  dbl_ovrd=off
  Counter : xbsIndex_r3/Counter  cnt_type=Free Running  n_bits=MaxDelay  bin_pt=0  arith_type=Unsigned  start_count=0  cnt_to=Inf  cnt_by_val=1  operation=Down  explicit_period=on  period=1  load_pin=on  rst=off  en=on  dbl_ovrd=off  show_param=off  use_rpm=on  gen_core=off
      settings: xl_area=[0, 0, 0, 0, 0, 0, 0]
  Logical : xbsIndex_r3/Logical  logical_function=OR  inputs=2  precision=Full  arith_type=Unsigned  n_bits=8  bin_pt=2  align_bp=on  latency=0  explicit_period=on  period=1  en=off  dbl_ovrd=off  show_param=off
      settings: xl_area=[0, 0, 0, 0, 0, 0, 0]
  Relational : xbsIndex_r3/Relational  mode=a=b  latency=0  explicit_period=off  period=1  en=off  dbl_ovrd=off  show_param=off
      settings: xl_area=[0, 0, 0, 0, 0, 0, 0]
  Relational1 : xbsIndex_r3/Relational  mode=a!=b  latency=0  explicit_period=on  period=1  en=off  dbl_ovrd=off  show_param=off
      settings: xl_area=[0, 0, 0, 0, 0, 0, 0]
  sync_out : Outport
  wires:
  Counter/1 -> Relational1/1, Relational/2
  Constant1/1 -> Relational1/2
  Constant/1 -> Relational/1
  delay/1 -> Counter/2
  sync/1 -> Counter/1, Logical/1
  Logical/1 -> Counter/3
  Relational1/1 -> Logical/2
  Relational/1 -> sync_out/1

== system casper_library/Downconverter/dds ==
  lo_const0 : casper_library/Downconverter/lo_const  n_bits=8  phase=0
  lo_const1 : casper_library/Downconverter/lo_const  n_bits=8  phase=1.5708
  lo_const2 : casper_library/Downconverter/lo_const  n_bits=8  phase=3.1416
  lo_const3 : casper_library/Downconverter/lo_const  n_bits=8  phase=4.7124
  sin0 : Outport
  cos0 : Outport  Port=2
  sin1 : Outport  Port=3
  cos1 : Outport  Port=4
  sin2 : Outport  Port=5
  cos2 : Outport  Port=6
  sin3 : Outport  Port=7
  cos3 : Outport  Port=8
  wires:
  lo_const0/1 -> sin0/1
  lo_const0/2 -> cos0/1
  lo_const1/1 -> sin1/1
  lo_const1/2 -> cos1/1
  lo_const2/1 -> sin2/1
  lo_const2/2 -> cos2/1
  lo_const3/1 -> sin3/1
  lo_const3/2 -> cos3/1

== system casper_library/Downconverter/dec_fir ==
  sync_in : Inport  Port=1  LatchInput=off
  real1 : Inport  Port=2  LatchInput=off
  imag1 : Inport  Port=3  LatchInput=off
  real2 : Inport  Port=4  LatchInput=off
  imag2 : Inport  Port=5  LatchInput=off
  real3 : Inport  Port=6  LatchInput=off
  imag3 : Inport  Port=7  LatchInput=off
  real4 : Inport  Port=8  LatchInput=off
  imag4 : Inport  Port=9  LatchInput=off
  convert1 : xbsIndex_r3/Convert  arith_type="Signed  (2's comp)"  n_bits=8  bin_pt=7  quantization=Truncate  overflow=Saturate  latency=2  explicit_period=on  period=1  dbl_ovrd=off  show_param=on  inserted_by_tool=off  pipeline=on
      settings: xl_area=[0, 0, 0, 0, 0, 0, 0]
  convert2 : xbsIndex_r3/Convert  arith_type="Signed  (2's comp)"  n_bits=8  bin_pt=7  quantization=Truncate  overflow=Saturate  latency=2  explicit_period=on  period=1  dbl_ovrd=off  show_param=on  inserted_by_tool=off  pipeline=on
      settings: xl_area=[0, 0, 0, 0, 0, 0, 0]
  delay : xbsIndex_r3/Delay  latency=5  reg_retiming=off  explicit_period=off  period=1  en=off  accept_only_valid=off  init_zero=on  dbl_ovrd=off  show_param=off
      settings: xl_area=[0, 0, 0, 0, 0, 0, 0]
  fir_col1 : Subsystem  AncestorBlock=casper_library/Downconverter/fir_col  mask(fir_col){n_inputs=4, coeff=[0.4 0.3 0.2 0.1], add_latency=2, mult_latency=2}
      mask prompts: n_inputs "Inputs"; coeff "Coefficients"; add_latency "Add latency"; mult_latency "Mult Latency"
      mask init:
      | fir_col_init(gcb, ...
      |     'n_inputs', n_inputs,...
      |     'coeff', coeff, ...
      |     'mult_latency', mult_latency, ...
      |     'add_latency', add_latency);
  imag_sum : Subsystem  AncestorBlock=casper_library/Misc/adder_tree  mask(adder_tree){n_inputs=1, latency=2}
      mask prompts: n_inputs "Number of Inputs"; latency "Add Latency"
      mask help: Sums all inputs using a tree of adds and delays.
      mask init:
      | adder_tree_init(gcb, ...
      |     'n_inputs', n_inputs, ...
      |     'latency', latency);
      settings: AttributesFormatString=latency 0
      mask Help: eval('xlWeb([getenv(''MLIB_ROOT''), ''\doc\html\sp_adder_tree\sp_adder_tree.html''])')
  real_sum : Subsystem  AncestorBlock=casper_library/Misc/adder_tree  mask(adder_tree){n_inputs=1, latency=2}
      mask prompts: n_inputs "Number of Inputs"; latency "Add Latency"
      mask help: Sums all inputs using a tree of adds and delays.
      mask init:
      | adder_tree_init(gcb, ...
      |     'n_inputs', n_inputs, ...
      |     'latency', latency);
      settings: AttributesFormatString=latency 0
      mask Help: eval('xlWeb([getenv(''MLIB_ROOT''), ''\doc\html\sp_adder_tree\sp_adder_tree.html''])')
  ri_to_c : Subsystem
  shift1 : xbsIndex_r3/Shift  shift_dir=Left  shift_bits=1  precision=Full  arith_type="Signed  (2's comp)"  n_bits=8  bin_pt=2  quantization=Truncate  overflow=Wrap  latency=0  explicit_period=off  period=1  en=off  dbl_ovrd=off  show_param=off
      settings: xl_area=[0, 0, 0, 0, 0, 0, 0]
  shift2 : xbsIndex_r3/Shift  shift_dir=Left  shift_bits=1  precision=Full  arith_type="Signed  (2's comp)"  n_bits=8  bin_pt=2  quantization=Truncate  overflow=Wrap  latency=0  explicit_period=off  period=1  en=off  dbl_ovrd=off  show_param=off
      settings: xl_area=[0, 0, 0, 0, 0, 0, 0]
  sync_out : Outport
  dout : Outport  Port=2
  wires:
  real1/1 -> fir_col1/1(real1)
  imag1/1 -> fir_col1/2(imag1)
  real2/1 -> fir_col1/3(real2)
  imag2/1 -> fir_col1/4(imag2)
  real3/1 -> fir_col1/5(real3)
  imag3/1 -> fir_col1/6(imag3)
  real4/1 -> fir_col1/7(real4)
  imag4/1 -> fir_col1/8(imag4)
  fir_col1/9(real_sum) -> real_sum/2(din1)
  fir_col1/10(imag_sum) -> imag_sum/2(din1)
  real_sum/2(dout) -> shift1/1
  imag_sum/2(dout) -> shift2/1
  shift1/1 -> convert1/1
  shift2/1 -> convert2/1
  convert1/1 -> ri_to_c/1(re)
  convert2/1 -> ri_to_c/2(im)
  ri_to_c/1(c) -> dout/1
  sync_in/1 -> delay/1
  delay/1 -> real_sum/1(sync), imag_sum/1(sync)
  real_sum/1(sync_out) -> sync_out/1

== system casper_library/Downconverter/fir_col ==
  real1 : Inport  Port=1  LatchInput=off
  imag1 : Inport  Port=2  LatchInput=off
  real2 : Inport  Port=3  LatchInput=off
  imag2 : Inport  Port=4  LatchInput=off
  adder_tree1 : Subsystem  AncestorBlock=casper_library/Misc/adder_tree  mask(adder_tree){n_inputs=2, latency=2}
      mask prompts: n_inputs "Number of Inputs"; latency "Add Latency"
      mask help: Sums all inputs using a tree of adds and delays.
      mask init:
      | adder_tree_init(gcb, ...
      |     'n_inputs', n_inputs, ...
      |     'latency', latency);
      settings: AttributesFormatString=latency 2
      mask Help: eval('xlWeb([getenv(''MLIB_ROOT''), ''\doc\html\sp_adder_tree\sp_adder_tree.html''])')
  adder_tree2 : Subsystem  AncestorBlock=casper_library/Misc/adder_tree  mask(adder_tree){n_inputs=2, latency=2}
      mask prompts: n_inputs "Number of Inputs"; latency "Add Latency"
      mask help: Sums all inputs using a tree of adds and delays.
      mask init:
      | adder_tree_init(gcb, ...
      |     'n_inputs', n_inputs, ...
      |     'latency', latency);
      settings: AttributesFormatString=latency 2
      mask Help: eval('xlWeb([getenv(''MLIB_ROOT''), ''\doc\html\sp_adder_tree\sp_adder_tree.html''])')
  c1 : xbsIndex_r3/Constant  const=1  equ=P=C  arith_type=Unsigned  n_bits=1  bin_pt=0  opselect=C  inp2=PCIN>>17  opr=+  inp1=P  carry=CIN  iostate=0  explicit_period=off  period=1  dbl_ovrd=off
  c2 : xbsIndex_r3/Constant  const=1  equ=P=C  arith_type=Unsigned  n_bits=1  bin_pt=0  opselect=C  inp2=PCIN>>17  opr=+  inp1=P  carry=CIN  iostate=0  explicit_period=off  period=1  dbl_ovrd=off
  fir_tap1 : Subsystem  AncestorBlock=casper_library/Downconverter/fir_tap  mask(fir_tap){factor=0.1, latency=2}
      mask prompts: latency "Mult latency"
  fir_tap2 : Subsystem  AncestorBlock=casper_library/Downconverter/fir_tap  mask(fir_tap){factor=0.2, latency=2}
      mask prompts: latency "Mult latency"
  real_out1 : Outport
  imag_out1 : Outport  Port=2
  real_out2 : Outport  Port=3
  imag_out2 : Outport  Port=4
  real_sum : Outport  Port=5
  imag_sum : Outport  Port=6
  wires:
  c1/1 -> adder_tree1/1(sync)
  c2/1 -> adder_tree2/1(sync)
  adder_tree1/2(dout) -> real_sum/1
  adder_tree2/2(dout) -> imag_sum/1
  real1/1 -> fir_tap1/1(a)
  imag1/1 -> fir_tap1/2(b)
  fir_tap1/1(a_out) -> real_out1/1
  fir_tap1/2(b_out) -> imag_out1/1
  fir_tap1/3(real) -> adder_tree1/2(din1)
  fir_tap1/4(imag) -> adder_tree2/2(din1)
  real2/1 -> fir_tap2/1(a)
  imag2/1 -> fir_tap2/2(b)
  fir_tap2/1(a_out) -> real_out2/1
  fir_tap2/2(b_out) -> imag_out2/1
  fir_tap2/3(real) -> adder_tree1/3(din2)
  fir_tap2/4(imag) -> adder_tree2/3(din2)
